simulink model "sfc"  (R2021a)
settings: Solver=VariableStepAuto  StartTime=0.0  StopTime=10.0  RelTol=1e-3
undefined symbols (not defined in the file or in its folder): A, B, C, D, K, x0
settings Model: Creator=itama  LastModifiedBy=itama

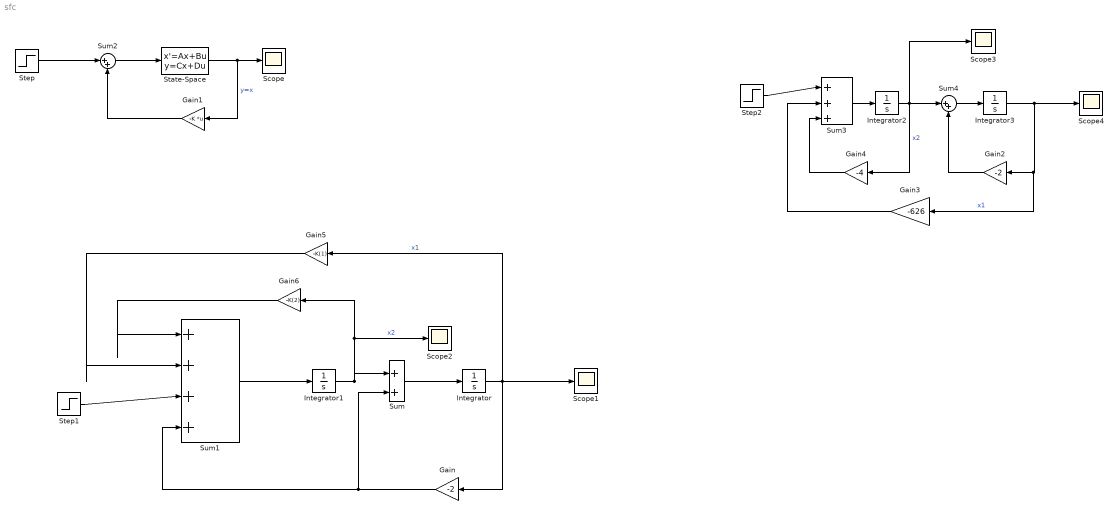
== system sfc ==
  Gain : Gain  Gain=-2
  Gain1 : Gain  Gain=-K  Multiplication=Matrix(K*u)
  Gain2 : Gain  Gain=-2
  Gain3 : Gain  Gain=-626
  Gain4 : Gain  Gain=-4
  Gain5 : Gain  Gain=-K(1)
  Gain6 : Gain  Gain=-K(2)
  Integrator{,1..3} (4 alike) : Integrator
  Scope{,1..4} (5 alike) : Scope
  State-Space : StateSpace  A=A  B=B  C=C  D=D  InitialCondition=x0
  Step : Step  SampleTime=0
  Step1 : Step  SampleTime=0
  Step2 : Step  SampleTime=0
  Sum : Sum  Inputs=|++
  Sum1 : Sum  Inputs=|++++
  Sum2 : Sum  Inputs=|++
  Sum3 : Sum  Inputs=|+++
  Sum4 : Sum  Inputs=|++
  wires:
  Sum4/1 -> Integrator3/1
  Gain/1 -> Sum1/4, Sum/2
  Sum2/1 -> State-Space/1
  Integrator3/1 -> Gain3/1, Gain2/1, Scope4/1  "x1"
  Gain2/1 -> Sum4/2
  Gain6/1 -> Sum1/1
  Gain4/1 -> Sum3/3
  Step1/1 -> Sum1/3
  Step/1 -> Sum2/1
  Sum/1 -> Integrator/1
  Step2/1 -> Sum3/1
  State-Space/1 -> Gain1/1, Scope/1  "y=x"
  Gain5/1 -> Sum1/2
  Integrator/1 -> Gain5/1, Gain/1, Scope1/1  "x1"
  Sum3/1 -> Integrator2/1
  Sum1/1 -> Integrator1/1
  Integrator1/1 -> Sum/1, Gain6/1, Scope2/1  "x2"
  Gain1/1 -> Sum2/2
  Gain3/1 -> Sum3/2
  Integrator2/1 -> Gain4/1, Scope3/1, Sum4/1  "x2"
